simulink model "Car_Wiper_MiL_Testing_by_NV_PATEL"  (R2022a)
settings: Solver=FixedStepDiscrete  StartTime=0.0  StopTime=0.5  FixedStep=0.1  MaxStep=0.1  RelTol=1e-3
undefined symbols (not defined in the file): sigbuilder_block
settings Model: Creator=jamesbond  LastModifiedBy=jamesbond
settings OptimizationCC: ZeroExternalMemoryAtStartup=off  ZeroInternalMemoryAtStartup=off
settings HardwareCC: ProdBitPerLong=64  ProdLongLongMode=on  ProdHWDeviceType=Intel->x86-64 (Mac OS X)
settings RTWCC: GenCodeOnly=on  TargetLang=C++
settings GRTTargetCC: TargetLangStandard=C++11 (ISO)  CodeInterfacePackaging=C++ class
settings ConfigComp: CovEnable=on  CovScope=ReferencedModels  CovIncludeTopModel=off  CovModelRefEnable=filtered

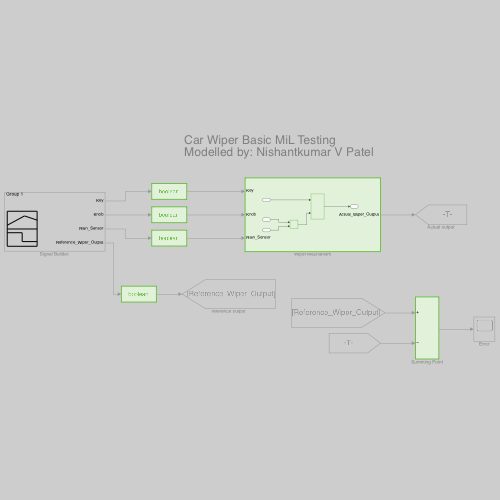
[thumbnail: Simulink's stored preview of the top-level diagram]
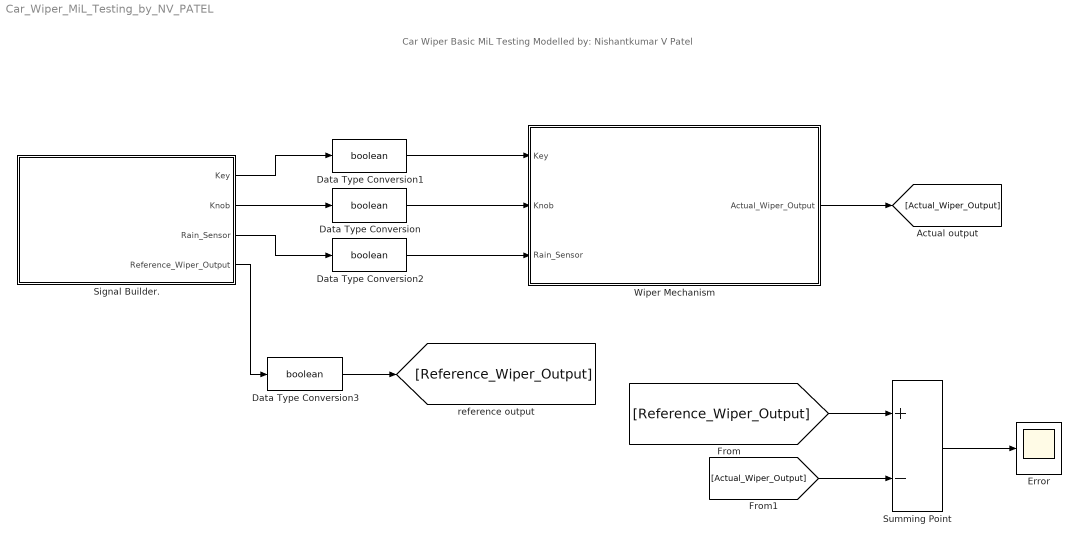
== system Car_Wiper_MiL_Testing_by_NV_PATEL ==
  note: Car Wiper Basic MiL Testing
      | Modelled by: Nishantkumar V Patel
  Data Type Conversion{,1..3} (4 alike) : DataTypeConversion  OutDataTypeStr=boolean  SaturateOnIntegerOverflow=off  RndMeth=Floor
  Error : Scope
  Signal Builder. : Subsystem  Tag=STV Subsys  LoadFcn=sigbuilder_block('load');  StartFcn=sigbuilder_block('start');  StopFcn=sigbuilder_block('stop');  ClipboardFcn=sigbuilder_block('clipboard');  mask(Sigbuilder block){tuvar=[0:10]}
      mask help: Simulink:masks:SigbuilderBlock_MD
      mask init:
      | if ~strcmp(get_param(bdroot(gcbh),'SimulationStatus'),'stopped') tuvar = sigbuilder_block('maskInit'); end
      settings: CopyFcn=sigbuilder_block('copy');  DeleteFcn=sigbuilder_block('delete');  ModelCloseFcn=sigbuilder_block('modelClose');  PreSaveFcn=sigbuilder_block('preSave');  PauseFcn=sigbuilder_block('pause');  ContinueFcn=sigbuilder_block('continue');  NameChangeFcn=sigbuilder_block('namechange');  OpenFcn=sigbuilder_block('open',[179 117 628 527 ]);  CloseFcn=sigbuilder_block('close');
      mask Display: plot(0, 0, 100, 100,[2, 2, 32, 32, 2], [68, 8, 8, 68, 68],[32, 2], [38, 38], [32, 19, 2],[53, 60, 44], [32, 17, 17, 2],[16, 16, 31, 31]);txt = getActiveGroup(gcbh);text(2, 100, txt,'verticalAlignment', 'top');
  Summing Point : Sum  Inputs=+-
  Wiper Mechanism : Subsystem
  wires:
  Signal Builder./1(Key) -> Data Type Conversion1/1
  Signal Builder./2(Knob) -> Data Type Conversion/1
  Signal Builder./3(Rain_Sensor) -> Data Type Conversion2/1
  Summing Point/1 -> Error/1
  [Reference_Wiper_Output] -> Summing Point/1
  Wiper Mechanism/1(Actual_Wiper_Output) -> [Actual_Wiper_Output]
  [Actual_Wiper_Output] -> Summing Point/2
  Data Type Conversion1/1 -> Wiper Mechanism/1(Key)
  Data Type Conversion/1 -> Wiper Mechanism/2(Knob)
  Data Type Conversion2/1 -> Wiper Mechanism/3(Rain_Sensor)
  Data Type Conversion3/1 -> [Reference_Wiper_Output]
  Signal Builder./4(Reference_Wiper_Output) -> Data Type Conversion3/1

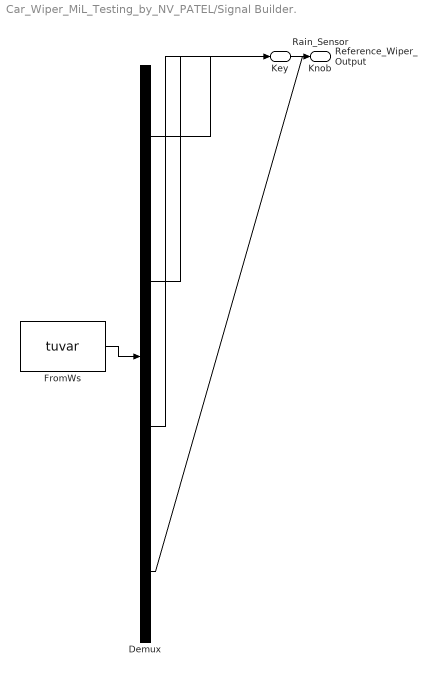
== system Car_Wiper_MiL_Testing_by_NV_PATEL/Signal Builder. ==
  Demux : Demux  Tag=STV Demux
      settings: DisplayOption=none
  FromWs : FromWorkspace  Tag=STV FromWs  VariableName=tuvar
      SigBuilderData=|
      | common.afterFinalStr = 'Extrapolate'
      | common.sampleTime = 0
      | dataSet.timeRange = [0 0.5]
      | dataSet.name = 'Group 1'
      | sbobj.Groups.Name = 'Group 1'
      | sbobj.Groups.Signals(1).Name = 'Key'
      | sbobj.Groups.Signals(1).XData = [0 0.1 0.2 0.3 0.4 0.5]
      | sbobj.Groups.Signals(1).YData = [0 1 1 1 1 0.01]
      | sbobj.Groups.Signals(2).Name = 'Knob'
      | sbobj.Groups.Signals(2).XData = [0 0.1 0.1005 0.2 0.3005 0.4 0.4 0.5]
      | sbobj.Groups.Signals(2).YData = [0 1 1 0 1 -0.01 0 1]
      | sbobj.Groups.Signals(3).Name = 'Rain_Sensor'
      | sbobj.Groups.Signals(3).XData = [0 0.1 0.2 0.3 0.4005 0.5]
      | sbobj.Groups.Signals(3).YData = [0 0 1 1 0 1]
      | sbobj.Groups.Signals(4).Name = 'Reference_Wiper_Output'
      | sbobj.Groups.Signals(4).XData = [0 0.1005 0.2 0.3 0.4 0.5]
      | sbobj.Groups.Signals(4).YData = [0 1 1 1 0 0]
      | sbobj.Groups.TimeRange = [0 0.5]
  Key : Outport  Tag=STV Outport
  Knob : Outport  Tag=STV Outport  Port=2
  Rain_Sensor : Outport  Tag=STV Outport  Port=3
  Reference_Wiper_Output : Outport  Tag=STV Outport  Port=4
  wires:
  FromWs/1 -> Demux/1
  Demux/1 -> Key/1
  Demux/2 -> Knob/1
  Demux/3 -> Rain_Sensor/1
  Demux/4 -> Reference_Wiper_Output/1

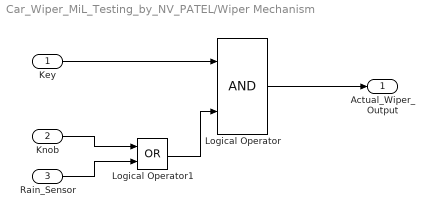
== system Car_Wiper_MiL_Testing_by_NV_PATEL/Wiper Mechanism ==
  Key : Inport
  Knob : Inport  Port=2
  Rain_Sensor : Inport  Port=3
  Logical Operator : Logic  AllPortsSameDT=off  OutDataTypeStr=boolean
  Logical Operator1 : Logic  Operator=OR  AllPortsSameDT=off  OutDataTypeStr=boolean
  Actual_Wiper_Output : Outport
  wires:
  Knob/1 -> Logical Operator1/1
  Logical Operator/1 -> Actual_Wiper_Output/1
  Rain_Sensor/1 -> Logical Operator1/2
  Key/1 -> Logical Operator/1
  Logical Operator1/1 -> Logical Operator/2
